simulink model "aprenfinal"  (Simulink 3.00)
settings: Solver=ode45  SolverMode=SingleTasking  StartTime=0.0  StopTime=2.5  FixedStep=0.01  RelTol=1e-3  AbsTol=1e-6
libraries: HEMERO x4
settings Model: OutputTimes=[1,2]  LastModifiedBy=Administrador

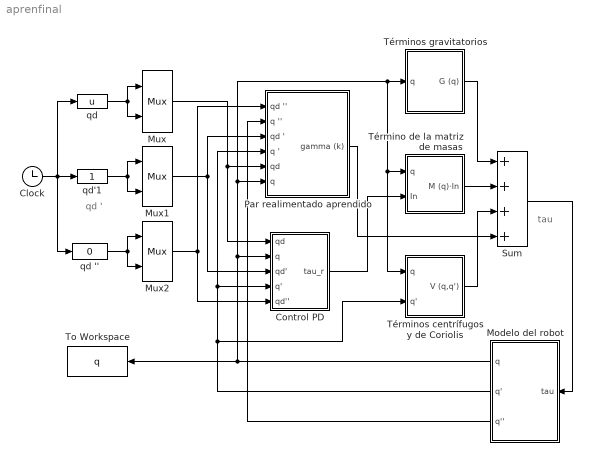
== system aprenfinal ==
  note: tau
  note: qd '
  Clock : Clock
      settings: DisplayTime=off  Decimation=10
  Control PD : Subsystem  mask(Controlador PD){Kp=[625 0;0 625], Kv=[50 0;0 50]}
      mask prompts: Kp "Introduzca la matriz Kp:"; Kv "Introduzca la matriz Kv:"
      mask help: Calcula el par tau_r correspondiente a la técnica del par computado usando un controlador PD.
  Modelo del robot : Subsystem  Orientation=left  mask(Trayectorias articulares){dyn=[0 0 0 0 0 0.8 1 0 0 0 0 0 0 0 0 0 1 10 0 0;0 1 0 0 0 2.3 1 0 0 0 0 0 0 0 0 0 1 5 0 0], grav=[0 -9.81 0], inivel=[0 0], inipos=[0 0]}
      mask prompts: dyn "Matriz de parámetros cinemáticos y dinámicos:"; grav "Vector aceleración de la gravedad:"; inivel "Velocidades articulares iniciales:"; inipos "Posiciones articulares iniciales:"
      mask help: Se calculan las trayectorias articulares (posiciones, velocidades y aceleraciones articulares) a partir de los pares aplicados al manipulador.
  Mux : Mux  Inputs=2
      settings: DisplayOption=none
  Mux1 : Mux  Inputs=2
      settings: DisplayOption=none
  Mux2 : Mux  Inputs=2
      settings: DisplayOption=none
  Par realimentado aprendido : Subsystem  mask{dyn=[0 0 0 0 0 0.8 1 0 0 0 0 0 0 0 0 0 1 0 0 0;0 1 0 0 0 2.3 1 0 0 0 0 0 0 0 0 0 1 0 0 0], Kp=625*eye(2), Kv=50*eye(2), mu=[3 0; 0 3], tfinal=2.5}
      mask prompts: dyn "Matriz de parámetros cinemáticos y dinámicos:"; Kp "Matriz Kp:"; Kv "Matriz Kv:"; mu "Constante mu:"; tfinal "Tiempo final de la simulación:"
  Sum : Sum  Inputs=++++  SaturateOnIntegerOverflow=on
  To Workspace : ToWorkspace  VariableName=q  SampleTime=-1  SaveFormat=Matrix
  Término de la matriz de masas : Subsystem  mask(Término asociado a la matriz de masas){dyn=[0 0 0 0 0 0.8 1 0 0 0 0 0 0 0 0 0 1 0 0 0;0 1 0 0 0 2.3 1 0 0 0 0 0 0 0 0 0 1 0 0 0]}
      mask prompts: dyn "Matriz de parámetros cinemáticos y dinámicos:"
      mask help: Este bloque calcula el par correspondiente al término en el que aparece la matriz de masas.
  Términos gravitatorios : Subsystem  mask(Término gravitatorio){dyn=[0 0 0 0 0 0.8 1 0 0 0 0 0 0 0 0 0 1 0 0 0;0 1 0 0 0 2.3 1 0 0 0 0 0 0 0 0 0 1 0 0 0], grav=[0 -9.81 0]}
      mask prompts: dyn "Matriz de parámetros cinemáticos y dinámicos:"; grav "Vector aceleración de la gravedad:"
      mask help: Este bloque calcula el par correspondiente al término gravitatorio.
  Términos centrífugos y de Coriolis : Subsystem  mask(Términos centrífugos y de Coriolis){dyn=[0 0 0 0 0 0.8 1 0 0 0 0 0 0 0 0 0 1 0 0 0;0 1 0 0 0 2.3 1 0 0 0 0 0 0 0 0 0 1 0 0 0]}
      mask prompts: dyn "Matriz de parámetros cinemáticos y dinámicos:"
      mask help: Este bloque calcula el par correspondiente a los términos centrífugos y de Coriolis.
  qd : Fcn  Expr=u
  qd '' : Fcn  Expr=0
  qd'1 : Fcn  Expr=1
  wires:
  Mux/1 -> Control PD/1(qd), Par realimentado aprendido/5(qd)
  Clock/1 -> qd/1, qd'1/1, qd ''/1
  Mux2/1 -> Control PD/5(qd''), Par realimentado aprendido/1(qd '')
  Mux1/1 -> Control PD/3(qd'), Par realimentado aprendido/3(qd ')
  qd/1 -> Mux/1, Mux/2
  qd'1/1 -> Mux1/1, Mux1/2
  qd ''/1 -> Mux2/1, Mux2/2
  Término de la matriz de masas/1(M (q)·In) -> Sum/2
  Términos centrífugos y de Coriolis/1(V (q,q')) -> Sum/3
  Términos gravitatorios/1(G (q)) -> Sum/1
  Control PD/1(tau_r) -> Término de la matriz de masas/2(In)
  Modelo del robot/2(q') -> Términos centrífugos y de Coriolis/2(q'), Control PD/4(q'), Par realimentado aprendido/4(q ')
  Modelo del robot/1(q) -> To Workspace/1, Control PD/2(q), Par realimentado aprendido/6(q), Términos centrífugos y de Coriolis/1(q), Término de la matriz de masas/1(q), Términos gravitatorios/1(q)
  Modelo del robot/3(q'') -> Par realimentado aprendido/2(q '')
  Sum/1 -> Modelo del robot/1(tau)
  Par realimentado aprendido/1(gamma (k)) -> Sum/4

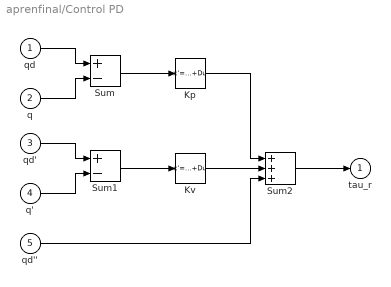
== system aprenfinal/Control PD ==
  qd : Inport  Port=1  PortWidth=-1  SampleTime=-1  DataType=auto
      settings: SignalType=auto
  q : Inport  Port=2  PortWidth=-1  SampleTime=-1  DataType=auto
      settings: SignalType=auto
  qd' : Inport  Port=3  PortWidth=-1  SampleTime=-1  DataType=auto
      settings: SignalType=auto
  q' : Inport  Port=4  PortWidth=-1  SampleTime=-1  DataType=auto
      settings: SignalType=auto
  qd'' : Inport  Port=5  PortWidth=-1  SampleTime=-1  DataType=auto
      settings: SignalType=auto
  Kp : StateSpace  A=[]  B=[]  C=[]  D=K  X0=0  mask(Matrix Gain){@1=Kp}
      mask prompts: @1 "Gain matrix:"
      mask help: Matrix Gain.
      mask init:
      | K=@1;
      mask Help: Multiplies input vector by entered matrix to produce output vector (y=Au).
      mask Display: disp('K')
  Kv : StateSpace  A=[]  B=[]  C=[]  D=K  X0=0  mask(Matrix Gain){@1=Kv}
      mask prompts: @1 "Gain matrix:"
      mask help: Matrix Gain.
      mask init:
      | K=@1;
      mask Help: Multiplies input vector by entered matrix to produce output vector (y=Au).
      mask Display: disp('K')
  Sum : Sum  Inputs=+-  SaturateOnIntegerOverflow=on
  Sum1 : Sum  Inputs=+-  SaturateOnIntegerOverflow=on
  Sum2 : Sum  Inputs=+++  SaturateOnIntegerOverflow=on
  tau_r : Outport  Port=1  InitialOutput=0
  wires:
  Sum2/1 -> tau_r/1
  qd''/1 -> Sum2/3
  Kp/1 -> Sum2/1
  Kv/1 -> Sum2/2
  Sum1/1 -> Kv/1
  Sum/1 -> Kp/1
  q'/1 -> Sum1/2
  qd'/1 -> Sum1/1
  q/1 -> Sum/2
  qd/1 -> Sum/1

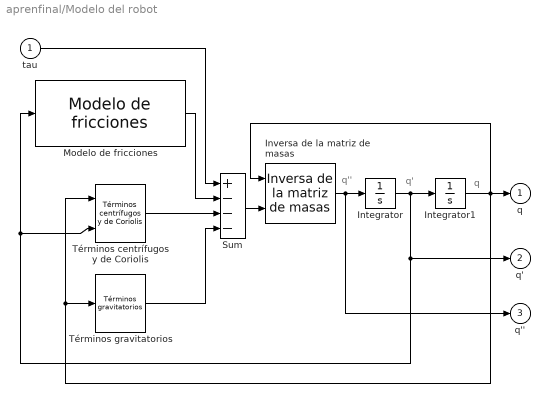
== system aprenfinal/Modelo del robot ==
  note: q
  note: q''
  note: q'
  tau : Inport  Port=1  PortWidth=-1  SampleTime=-1  DataType=auto
      settings: SignalType=auto
  Integrator : Integrator  ExternalReset=none  InitialConditionSource=internal  InitialCondition=inivel(:)  LimitOutput=off  UpperSaturationLimit=inf  LowerSaturationLimit=-inf  ShowSaturationPort=off  ShowStatePort=off  AbsoluteTolerance=auto
  Integrator1 : Integrator  ExternalReset=none  InitialConditionSource=internal  InitialCondition=inipos(:)  LimitOutput=off  UpperSaturationLimit=inf  LowerSaturationLimit=-inf  ShowSaturationPort=off  ShowStatePort=off  AbsoluteTolerance=auto
  Inversa de la matriz de masas : HEMERO/Robots manipuladores base fija/Modelo Dinámico/Trayectorias articulares/Inversa de la matriz de masas  dyn=dyn
  Modelo de fricciones : HEMERO/Robots manipuladores base fija/Modelo Dinámico/Trayectorias articulares/Modelo de fricciones  G=dyn (:,17)  b=dyn (:,18)  tcp=dyn (:,19)  tcm=dyn (:,20)
  Sum : Sum  Inputs=+---  SaturateOnIntegerOverflow=on
  Términos gravitatorios : HEMERO/Robots manipuladores base fija/Modelo Dinámico/Trayectorias articulares/Términos gravitatorios  dyn=dyn  grav=grav
  Términos centrífugos y de Coriolis : HEMERO/Robots manipuladores base fija/Modelo Dinámico/Trayectorias articulares/Términos centrífugos y de Coriolis  dyn=dyn
  q : Outport  Port=1  InitialOutput=0
  q' : Outport  Port=2  InitialOutput=0
  q'' : Outport  Port=3  InitialOutput=0
  wires:
  Integrator1/1 -> q/1, Inversa de la matriz de masas/1, Términos centrífugos y de Coriolis/1, Términos gravitatorios/1
  Integrator/1 -> Integrator1/1, q'/1, Términos centrífugos y de Coriolis/2, Modelo de fricciones/1
  Sum/1 -> Inversa de la matriz de masas/2
  tau/1 -> Sum/1
  Inversa de la matriz de masas/1 -> Integrator/1, q''/1
  Términos gravitatorios/1 -> Sum/4
  Términos centrífugos y de Coriolis/1 -> Sum/3
  Modelo de fricciones/1 -> Sum/2

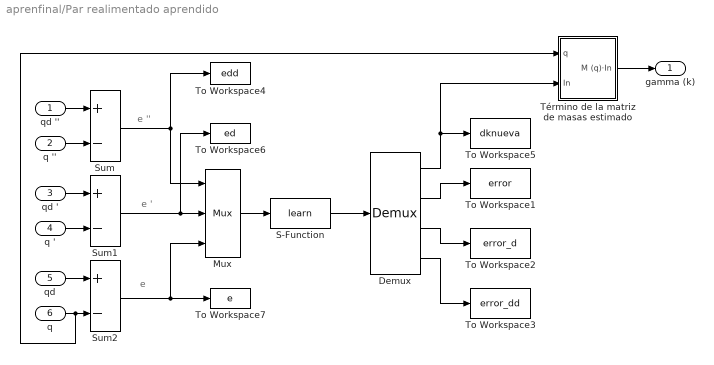
== system aprenfinal/Par realimentado aprendido ==
  note: e ''
  note: e '
  note: e
  qd '' : Inport  Port=1  PortWidth=-1  SampleTime=-1  DataType=auto
      settings: SignalType=auto
  q '' : Inport  Port=2  PortWidth=-1  SampleTime=-1  DataType=auto
      settings: SignalType=auto
  qd ' : Inport  Port=3  PortWidth=-1  SampleTime=-1  DataType=auto
      settings: SignalType=auto
  q ' : Inport  Port=4  PortWidth=-1  SampleTime=-1  DataType=auto
      settings: SignalType=auto
  qd : Inport  Port=5  PortWidth=-1  SampleTime=-1  DataType=auto
      settings: SignalType=auto
  q : Inport  Port=6  PortWidth=-1  SampleTime=-1  DataType=auto
      settings: SignalType=auto
  Demux : Demux  Outputs=4
  Mux : Mux  Inputs=3
      settings: DisplayOption=none
  S-Function : S-Function  FunctionName=learn  Parameters=Kp, Kv, mu, tfinal  PortCounts=[]  SFunctionModules=''
  Sum : Sum  Inputs=+-  SaturateOnIntegerOverflow=on
  Sum1 : Sum  Inputs=+-  SaturateOnIntegerOverflow=on
  Sum2 : Sum  Inputs=+-  SaturateOnIntegerOverflow=on
  To Workspace1 : ToWorkspace  VariableName=error  SampleTime=-1  SaveFormat=Matrix
  To Workspace2 : ToWorkspace  VariableName=error_d  SampleTime=-1  SaveFormat=Matrix
  To Workspace3 : ToWorkspace  VariableName=error_dd  SampleTime=-1  SaveFormat=Matrix
  To Workspace4 : ToWorkspace  VariableName=edd  SampleTime=-1  SaveFormat=Matrix
  To Workspace5 : ToWorkspace  VariableName=dknueva  SampleTime=-1  SaveFormat=Matrix
  To Workspace6 : ToWorkspace  VariableName=ed  SampleTime=-1  SaveFormat=Matrix
  To Workspace7 : ToWorkspace  VariableName=e  SampleTime=-1  SaveFormat=Matrix
  Término de la matriz de masas estimado : Subsystem  mask(Término asociado a la matriz de masas){dyn=dyn}
      mask prompts: dyn "Matriz de parámetros cinemáticos y dinámicos:"
      mask help: Este bloque calcula el par correspondiente al término en el que aparece la matriz de masas.
  gamma (k) : Outport  Port=1
  wires:
  Mux/1 -> S-Function/1
  S-Function/1 -> Demux/1
  qd ''/1 -> Sum/1
  q ''/1 -> Sum/2
  qd '/1 -> Sum1/1
  q '/1 -> Sum1/2
  qd/1 -> Sum2/1
  Demux/1 -> Término de la matriz de masas estimado/2(In), To Workspace5/1
  Sum2/1 -> Mux/3, To Workspace7/1
  Sum1/1 -> Mux/2, To Workspace6/1
  Sum/1 -> Mux/1, To Workspace4/1
  Demux/2 -> To Workspace1/1
  Demux/3 -> To Workspace2/1
  Demux/4 -> To Workspace3/1
  q/1 -> Sum2/2, Término de la matriz de masas estimado/1(q)
  Término de la matriz de masas estimado/1(M (q)·In) -> gamma (k)/1

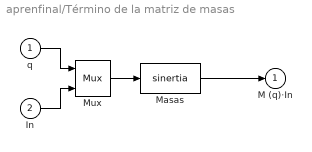
== system aprenfinal/Término de la matriz de masas ==
  q : Inport  Port=1  PortWidth=-1  SampleTime=-1  DataType=auto
      settings: SignalType=auto
  In : Inport  Port=2  PortWidth=-1  SampleTime=-1  DataType=auto
      settings: SignalType=auto
  Masas : S-Function  FunctionName=sinertia  Parameters=dyn  PortCounts=[]  SFunctionModules=''
  Mux : Mux  Inputs=2
      settings: DisplayOption=none
  M (q)·In : Outport  Port=1  InitialOutput=0
  wires:
  Masas/1 -> M (q)·In/1
  In/1 -> Mux/2
  q/1 -> Mux/1
  Mux/1 -> Masas/1

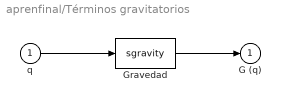
== system aprenfinal/Términos gravitatorios ==
  q : Inport  Port=1  PortWidth=-1  SampleTime=-1  DataType=auto
      settings: SignalType=auto
  Gravedad : S-Function  FunctionName=sgravity  Parameters=dyn,grav  PortCounts=[]  SFunctionModules=''
  G (q) : Outport  Port=1  InitialOutput=0
  wires:
  Gravedad/1 -> G (q)/1
  q/1 -> Gravedad/1

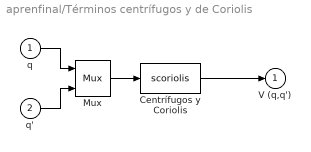
== system aprenfinal/Términos centrífugos y de Coriolis ==
  q : Inport  Port=1  PortWidth=-1  SampleTime=-1  DataType=auto
      settings: SignalType=auto
  q' : Inport  Port=2  PortWidth=-1  SampleTime=-1  DataType=auto
      settings: SignalType=auto
  Centrífugos y Coriolis : S-Function  FunctionName=scoriolis  Parameters=dyn  PortCounts=[]  SFunctionModules=''
  Mux : Mux  Inputs=2
      settings: DisplayOption=none
  V (q,q') : Outport  Port=1  InitialOutput=0
  wires:
  Centrífugos y Coriolis/1 -> V (q,q')/1
  q'/1 -> Mux/2
  q/1 -> Mux/1
  Mux/1 -> Centrífugos y Coriolis/1

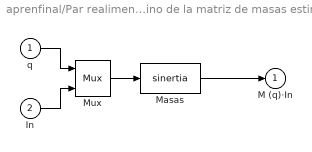
== system aprenfinal/Par realimentado aprendido/Término de la matriz de masas estimado ==
  q : Inport  Port=1  PortWidth=-1  SampleTime=-1  DataType=auto
      settings: SignalType=auto
  In : Inport  Port=2  PortWidth=-1  SampleTime=-1  DataType=auto
      settings: SignalType=auto
  Masas : S-Function  FunctionName=sinertia  Parameters=dyn  PortCounts=[]  SFunctionModules=''
  Mux : Mux  Inputs=2
      settings: DisplayOption=none
  M (q)·In : Outport  Port=1  InitialOutput=0
  wires:
  Masas/1 -> M (q)·In/1
  In/1 -> Mux/2
  q/1 -> Mux/1
  Mux/1 -> Masas/1
